simulink model "simulink_PD_controller"  (R2023a)
settings: Solver=VariableStepAuto  StartTime=0.0  StopTime=389  RelTol=1e-8
libraries: simulink x3
settings Model: Creator=ganes  LastModifiedBy=ganes

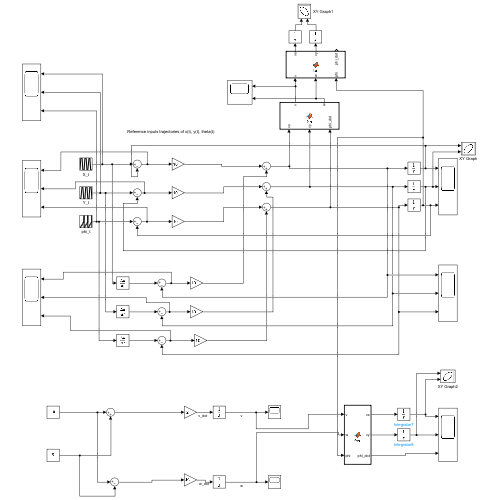
[thumbnail: Simulink's stored preview of the top-level diagram]
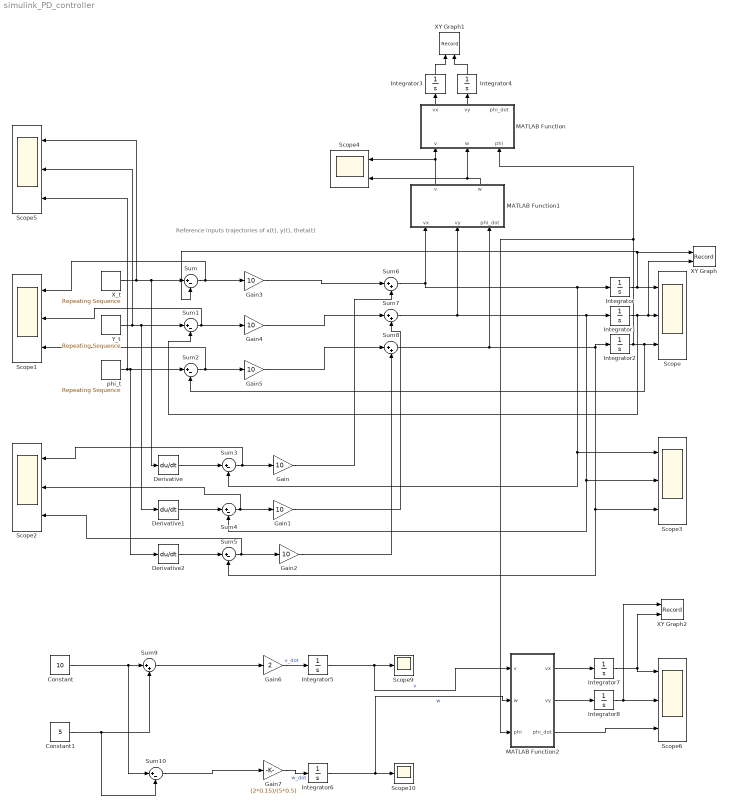
== system simulink_PD_controller ==
  note: Reference inputs trajectories of x(t), y(t), theta(t)
  Constant : Constant  Value=10
  Constant1 : Constant  Value=5
  Derivative : Derivative
  Derivative1 : Derivative
  Derivative2 : Derivative
  Gain{,1..5} (6 alike) : Gain  Gain=10
  Gain6 : Gain  Gain=2
  Gain7 : Gain  Gain=(2*0.15)/(5*0.5)
  Integrator{,1..8} (9 alike) : Integrator
  MATLAB Function : MATLAB Function  TreatAsAtomicUnit=on
  MATLAB Function1 : MATLAB Function  TreatAsAtomicUnit=on
  MATLAB Function2 : MATLAB Function  TreatAsAtomicUnit=on
  Scope{,1..3,5..6} (6 alike) : Scope  NumInputPorts=3
  Scope10 : Scope
  Scope4 : Scope  NumInputPorts=2
  Scope9 : Scope
  Sum{,1..5,10} (7 alike) : Sum  Inputs=|+-
  Sum{6..9} (4 alike) : Sum  Inputs=|++
  XY Graph : Record  FileSettingsInternal="{\"entries\":[{\"content\":{\"excelSettings\":{\"content\":{},\"type\":\"Streamout.ExcelSettings\"}},\"type\":\"Streamout.FileSettingStorage\",\"uuid\":\"\"}],\"packageUris\":[\"http:\\/\\/schema.mathworks.com\\/mf0\\/streamout_blocks\\/R2020a\"],\"version\":\"1.0\"}"  Layout=[1 1]  SignalsInternal="{\"entries\":[{\"content\":{\"signals\":[{\"content\":{\"blockPath\":[],\"dimensions\":[1],\"domain\":\"\",\"lineColor\":\"#64d413\",\"port\":1,\"sid\":[\"\"],\"signalID\":923,\"signalName\":\"Integrator\"},\"type\":\"RecordBlkView.Signal\",\"uuid\":\"\"},{\"content\":{\"blockPath\":[],\"dimensions\":[1],\"domain\":\"\",\"lineColor\":\"#ff13a6\",\"port\":2,\"sid\":[\"\"],\"signalID\":927,\"signalName\":\"Integrator1\"},\"type\":\"RecordBlkView.Signal\",\"uuid\":\"\"}]},\"type\":\"RecordBlkView.InputSignals\",\"uuid\":\"\"}],\"packageUris\":[\"http:\\/\\/schema.mathworks.com\\/mf0\\/streamout_blocks\\/R2020a\"],\"version\":\"1.0\"}"  VisualizationBindings="{\"xyplotplugin\":{\"info\":[{\"series\":[],\"subplotID\":1}]}}"  CompatibilityTag=XY
  XY Graph1 : Record  FileSettingsInternal="{\"entries\":[{\"content\":{\"excelSettings\":{\"content\":{},\"type\":\"Streamout.ExcelSettings\"}},\"type\":\"Streamout.FileSettingStorage\",\"uuid\":\"\"}],\"packageUris\":[\"http:\\/\\/schema.mathworks.com\\/mf0\\/streamout_blocks\\/R2020a\"],\"version\":\"1.0\"}"  Layout=[1 1]  SignalsInternal="{\"entries\":[{\"content\":{\"signals\":[{\"content\":{\"blockPath\":[],\"dimensions\":[1],\"domain\":\"\",\"lineColor\":\"#fe330a\",\"plots\":[1],\"port\":1,\"sid\":[\"\"],\"signalID\":931,\"signalName\":\"Integrator3\"},\"type\":\"RecordBlkView.Signal\",\"uuid\":\"\"},{\"content\":{\"blockPath\":[],\"dimensions\":[1],\"domain\":\"\",\"lineColor\":\"#22b573\",\"port\":2,\"sid\":[\"\"],\"signalID\":935,\"signalName\":\"Integrator4\"},\"type\":\"RecordBlkView.Signal\",\"uuid\":\"\"}]},\"type\":\"RecordBlkView.InputSignals\",\"uuid\":\"\"}],\"packageUris\":[\"http:\\/\\/schema.mathworks.com\\/mf0\\/streamout_blocks\\/R2020a\"],\"version\":\"1.0\"}"  VisualizationBindings="{\"xyplotplugin\":{\"info\":[{\"series\":[{\"bindingParametersList\":[{\"parameter\":\"Y-Axis\",\"signalID\":931,\"signalName\":\"Integrator3\"}],\"seriesID\":58929}],\"subplotID\":1}]}}"  CompatibilityTag=XY
  XY Graph2 : Record  FileSettingsInternal="{\"entries\":[{\"content\":{\"excelSettings\":{\"content\":{},\"type\":\"Streamout.ExcelSettings\"}},\"type\":\"Streamout.FileSettingStorage\",\"uuid\":\"\"}],\"packageUris\":[\"http:\\/\\/schema.mathworks.com\\/mf0\\/streamout_blocks\\/R2020a\"],\"version\":\"1.0\"}"  Layout=[1 1]  SignalsInternal="{\"entries\":[{\"content\":{\"signals\":[{\"content\":{\"blockPath\":[],\"dimensions\":[1],\"domain\":\"\",\"lineColor\":\"#a2142f\",\"port\":1,\"sid\":[\"\"],\"signalID\":939,\"signalName\":\"Integrator8\"},\"type\":\"RecordBlkView.Signal\",\"uuid\":\"\"},{\"content\":{\"blockPath\":[],\"dimensions\":[1],\"domain\":\"\",\"lineColor\":\"#139fff\",\"plots\":[1],\"port\":2,\"sid\":[\"\"],\"signalID\":943,\"signalName\":\"Integrator7\"},\"type\":\"RecordBlkView.Signal\",\"uuid\":\"\"}]},\"type\":\"RecordBlkView.InputSignals\",\"uuid\":\"\"}],\"packageUris\":[\"http:\\/\\/schema.mathworks.com\\/mf0\\/streamout_blocks\\/R2020a\"],\"version\":\"1.0\"}"  VisualizationBindings="{\"xyplotplugin\":{\"info\":[{\"series\":[{\"bindingParametersList\":[{\"parameter\":\"Y-Axis\",\"signalID\":943,\"signalName\":\"Integrator7\"}],\"seriesID\":44514}],\"subplotID\":1}]}}"  CompatibilityTag=XY
  X_t : simulink/Sources/Repeating Sequence  rep_seq_t=t_vec  rep_seq_y=x_t
  Y_t : simulink/Sources/Repeating Sequence  rep_seq_t=t_vec  rep_seq_y=y_t
  phi_t : simulink/Sources/Repeating Sequence  rep_seq_t=t_vec  rep_seq_y=w
  wires:
  Sum7/1 -> Integrator1/1, Scope3/2, Sum4/2, MATLAB Function1/2(vy)
  Sum6/1 -> MATLAB Function1/1(vx), Scope3/1, Sum3/2, Integrator/1
  Integrator2/1 -> Scope/3, Sum2/2, MATLAB Function/3(phi), MATLAB Function2/3(phi)
  Integrator/1 -> Scope/1, Sum/2, XY Graph/1
  Integrator1/1 -> XY Graph/2, Scope/2, Sum1/2
  phi_t/1 -> Derivative2/1, Sum2/1, Scope5/3
  Y_t/1 -> Scope5/2, Derivative1/1, Sum1/1
  Derivative/1 -> Sum3/1
  Derivative1/1 -> Sum4/1
  Derivative2/1 -> Sum5/1
  Sum/1 -> Scope1/1, Gain3/1
  Sum1/1 -> Scope1/2, Gain4/1
  Sum3/1 -> Scope2/1, Gain/1
  Sum4/1 -> Scope2/2, Gain1/1
  Sum5/1 -> Scope2/3, Gain2/1
  Gain2/1 -> Sum8/2
  Gain1/1 -> Sum7/2
  Gain/1 -> Sum6/2
  Gain4/1 -> Sum7/1
  Gain5/1 -> Sum8/1
  Gain3/1 -> Sum6/1
  Sum2/1 -> Scope1/3, Gain5/1
  MATLAB Function1/1(v) -> MATLAB Function/1(v), Scope4/1
  MATLAB Function1/2(w) -> MATLAB Function/2(w), Scope4/2
  X_t/1 -> Scope5/1, Derivative/1, Sum/1
  MATLAB Function/1(vx) -> Integrator3/1
  MATLAB Function/2(vy) -> Integrator4/1
  Integrator3/1 -> XY Graph1/1
  Integrator4/1 -> XY Graph1/2
  Sum10/1 -> Gain7/1
  Constant/1 -> Sum10/1, Sum9/1
  Integrator5/1 -> MATLAB Function2/1(v), Scope9/1  "v"
  Gain6/1 -> Integrator5/1  "v_dot"
  Constant1/1 -> Sum10/2, Sum9/2
  Integrator6/1 -> Scope10/1, MATLAB Function2/2(w)  "w"
  MATLAB Function2/1(vx) -> Integrator7/1
  MATLAB Function2/2(vy) -> Integrator8/1
  Sum8/1 -> Integrator2/1, Scope3/3, Sum5/2, MATLAB Function1/3(phi_dot)
  MATLAB Function2/3(phi_dot) -> Scope6/3
  Integrator7/1 -> Scope6/1, XY Graph2/2
  Integrator8/1 -> XY Graph2/1, Scope6/2
  Sum9/1 -> Gain6/1
  Gain7/1 -> Integrator6/1  "w_dot"

== matlab function simulink_PD_controller/MATLAB Function1 ==
  data: vx input; v output; vy input; phi_dot input; w output
function [v, w] = fcn(vx, vy, phi_dot)
    v=sqrt(vx^2+vy^2);
    w=phi_dot;
end

== matlab function simulink_PD_controller/MATLAB Function ==
  data: v input; vx output; w input; phi input; vy output; phi_dot output
function [vx, vy, phi_dot] = fcn(v, w, phi)
    vx=v*cos(phi);
    vy=v*sin(phi);
    phi_dot=w;
end

== matlab function simulink_PD_controller/MATLAB Function2 ==
  data: v input; vx output; w input; vy output; phi input; phi_dot output
function [vx, vy, phi_dot] = fcn(v, w, phi)
    vx=v*cos(phi);
    vy=v*sin(phi);
    phi_dot=w;
end
